simulink model "EGPC"  (R2017a)
settings: Solver=ode4  StartTime=0.0  StopTime=10.0  FixedStep=0.1  RelTol=1e-3
settings Model: Creator=danielguerra  LastModifiedBy=danielguerra
settings SolverCC: AutoInsertRateTranBlk=on

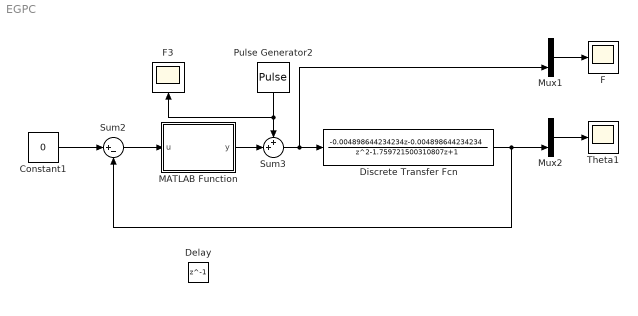
== system EGPC ==
  Constant1 : Constant  Value=0
  Delay : Delay  DelayLength=1
  Discrete Transfer Fcn : DiscreteTransferFcn  Numerator="[-0.004898644234234  -0.004898644234234]"  Denominator=[1 -1.759721500310807 1]
  F : Scope
  F3 : Scope
  MATLAB Function : MATLAB Function  TreatAsAtomicUnit=on
  Mux1 : Mux  Inputs=2
  Mux2 : Mux  Inputs=2
  Pulse Generator2 : DiscretePulseGenerator  PulseType=Time based  Period=20  PulseWidth=5
  Sum2 : Sum  Inputs=|+-
  Sum3 : Sum  Inputs=++|
  Theta1 : Scope
  wires:
  Mux1/1 -> F/1
  MATLAB Function/1(y) -> Sum3/2
  Constant1/1 -> Sum2/1
  Pulse Generator2/1 -> F3/1, Sum3/1
  Sum2/1 -> MATLAB Function/1(u)
  Sum3/1 -> Mux1/2, Discrete Transfer Fcn/1
  Mux2/1 -> Theta1/1
  Discrete Transfer Fcn/1 -> Mux2/2, Sum2/2

== matlab function EGPC/MATLAB Function ==
  data: u input; y output
function y = fcn(u)

y = u;
